simulink model "Model_1_with_driver"  (R2021a)
settings: Solver=VariableStepAuto  StartTime=0.0  StopTime=1561  RelTol=1e-3
model workspace (MATLAB code in the model file):
  | ms = 135;
  | mf = 5;
  | mr = 10;
  | m = ms + (mf + mr);
  | a = 0.7;
  | b = 0.7;
  | Cd = 0.8;
  | Af = 1;
  | h_cg = 0.5;
  | kf = 10000;
  | kr = 15000;
  | cf = 5000;
  | cr = 5000;
  | I = 500;
  | kt = 175000;
  | GR = 6.5;
  | Pmax = 5500;
  | Tmax = 26;
undefined symbols (not defined in the file or in its folder): bev
libraries: fl_lib x9, autolibshared x4, nesl_utility x3
(part 1 of 3)
settings Model: Creator=Barath Krishna S  LastModifiedBy=Ng
settings SolverCC: AlgebraicLoopSolver=TrustRegion
settings DebuggingCC: SFMachineParentedDataDiag=warning

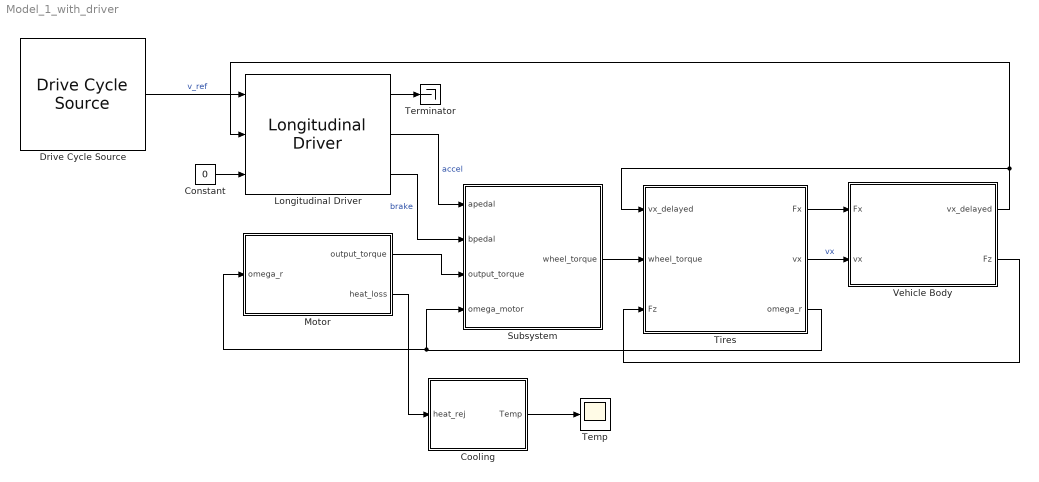
== system Model_1_with_driver ==
  Constant : Constant  Value=0
  Cooling : Subsystem
  Drive Cycle Source : autolibshared/Drive Cycle Source  cycleVar=Workspace variable  wsVar=mycycle  fileVar=cycleFTP75.mat  tfinal="1560.636  seconds"  cycleRepeat=off  outAccPort=off  outGearPort=off  gearList=No gear data  t_wot1=5  xdot_woto=0  xdot_wot1=30  t_wot2=20  xdot_wot2=0  t_wotend=30  srcUnit=m/s  outUnit=m/s  srcAccUnit=m/s/s  outAccUnit=m/s^2  dt=0  aMode=1  faultOption=off  velBnd=2  velBndUnit=mph  inUnit=m/s  timeBnd=1  failOption=off  stopSim=off  maxFaultCnt=10  maxFaultTime=2  maxTotFaultTime=15  traceOption=off  dtTrace=1  traceWindow=10  lastDCname=Custom Data Set  lastOutUnit=mph  lastDT=0  lastTB=1  lastSB=2  forceCalcBound=off
      settings: SourceProductBaseCode=PW,DR,MT,UV,VE
  Longitudinal Driver : autolibshared/Longitudinal Driver  extAccelOvr=off  extDecelOvr=off  extAccelHld=off  extDecelHld=off  extAccelZero=off  extDecelZero=off  cntrlType=PI  shftType=None  velUnits=m/s  gearOut=off  Kp=100  Ki=2.5  Kff=.05  Kg=.01  VehVelVec=[0 100]  KffVec=[.1 .1]  KpVec=[10 10]  KiVec=[5 5]  KgVec=[0 0]  m=1500  Kpt=3000  tau=.1  L=2  aR=200  bR=2.5  cR=.5  g=9.81  vnom=100  Kaw=.1  tauerr=.03  tauPt=2  GearInit=0  tShift=.1  pdlVec=[0.1 0.4 0.5 0.9]  upShftTbl=[-1 12.9375 26.4375 39.9375 51.18749999999999 62.4375 72.84375 83.25;-1 16.3125 29.8125 43.3125 54.5624 65.8125 76.78125 87.75;-1 19.6875 33.1875 46.68749999999999 57.9375 69.1875 80.71875 92.25;-1 33 52.5 77.25 100.5 138.75 161.875 185]  dwnShftTbl=[1 9.5625 23.0625 36.5625 47.8125 59.0625 68.90625 78.75;1 12.9375 26.4375 39.9375 51.18749999999999 62.4375 72.84375 83.25;1 16.3125 29.8125 43.3125 54.562499 65.8125 76.78125 87.75;1 19.6875 33.1875 46.68749999999999 57.9375 69.1875 80.71875 92.25]  tClutch=.5  tRev=.5  tPark=120  aMode=1  UpGearVec="[0  1  2  3  4  5  6  7]"  DownGearVec="[1  2  3  4  5  6  7  8]"
      settings: SourceProductBaseCode=PW,DR,MT,UV,VE
  Motor : Subsystem
  Subsystem : Subsystem
  Temp : Scope
  Terminator : Terminator
  Tires : Subsystem
  Vehicle Body : Subsystem
  wires:
  Tires/2(vx) -> Vehicle Body/2(vx)  "vx"
  Vehicle Body/2(Fz) -> Tires/3(Fz)
  Vehicle Body/1(vx_delayed) -> Longitudinal Driver/2, Tires/1(vx_delayed)
  Tires/1(Fx) -> Vehicle Body/1(Fx)
  Drive Cycle Source/1 -> Longitudinal Driver/1  "v_ref"
  Constant/1 -> Longitudinal Driver/3
  Longitudinal Driver/1 -> Terminator/1
  Longitudinal Driver/2 -> Subsystem/1(apedal)  "accel"
  Longitudinal Driver/3 -> Subsystem/2(bpedal)  "brake"
  Motor/1(output_torque) -> Subsystem/3(output_torque)
  Subsystem/1(wheel_torque) -> Tires/2(wheel_torque)
  Tires/3(omega_r) -> Subsystem/4(omega_motor), Motor/1(omega_r)
  Motor/2(heat_loss) -> Cooling/1(heat_rej)
  Cooling/1(Temp) -> Temp/1

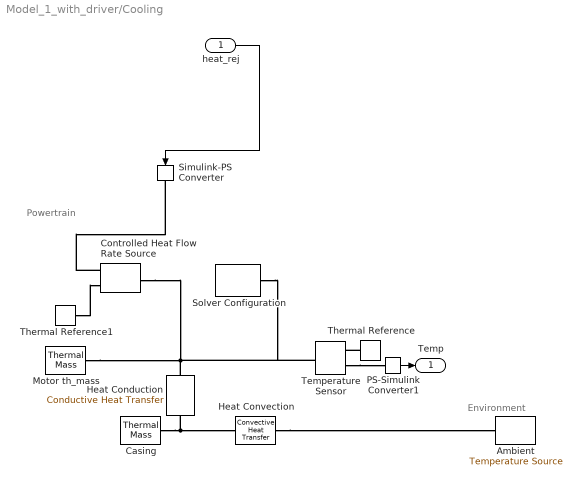
== system Model_1_with_driver/Cooling ==
  note: Powertrain
  note: Environment
  heat_rej : Inport
  Ambient : fl_lib/Thermal/Thermal Sources/Temperature Source  temperature=bev.Tambient degC
  Casing : fl_lib/Thermal/Thermal Elements/Thermal Mass  mass=bev.casing.mass kg  sp_heat=bev.casing.sp_heat J/kg/K  T_specify=on  T_priority=High  T=bev.casing.initT degC  T_nominal_specify=off  T_nominal_unit=K  T_nominal_value=1  Q_specify=off  Q_priority=None  Q=0 W  Q_nominal_specify=off  Q_nominal_unit=W  Q_nominal_value=1
  Controlled Heat Flow Rate Source : fl_lib/Thermal/Thermal Sources/Controlled Heat Flow Rate Source
  Heat Conduction : fl_lib/Thermal/Thermal Elements/Conductive Heat Transfer  area=bev.motor.qcond.area m^2  thickness=bev.motor.qcond.thick m  th_cond=bev.motor.qcond.th_cond W/(m*K)  T_specify=off  T_priority=None  T=0 K  T_nominal_specify=off  T_nominal_unit=K  T_nominal_value=1  Q_specify=off  Q_priority=None  Q=1 W  Q_nominal_specify=off  Q_nominal_unit=W  Q_nominal_value=1
  Heat Convection : fl_lib/Thermal/Thermal Elements/Convective Heat Transfer  area=bev.casing.qconv.area m^2  heat_tr_coeff=bev.casing.qconv.th_conv W/(m^2 * K)  T_specify=off  T_priority=None  T=0 K  T_nominal_specify=off  T_nominal_unit=K  T_nominal_value=1  Q_specify=off  Q_priority=None  Q=0 W  Q_nominal_specify=off  Q_nominal_unit=W  Q_nominal_value=1
  Motor th_mass : fl_lib/Thermal/Thermal Elements/Thermal Mass  mass=bev.motor.thermal_mass kg  sp_heat=1 J/kg/K  T_specify=on  T_priority=High  T=bev.motor.initT degC  T_nominal_specify=off  T_nominal_unit=K  T_nominal_value=1  Q_specify=off  Q_priority=None  Q=0 W  Q_nominal_specify=off  Q_nominal_unit=W  Q_nominal_value=1
  PS-Simulink Converter1 : nesl_utility/PS-Simulink Converter  PhysicalDomain=network_engine_domain  SubClassName=ps_output  LeftPortType=input  RightPortType=output  PseudoPeriodic=off  Frequencies=[]  Unit=degC  AffineConversion=on
      settings: SourceProductBaseCode=PW,SS
  Simulink-PS Converter : nesl_utility/Simulink-PS Converter  PhysicalDomain=network_engine_domain  SubClassName=ps_input  LeftPortType=input  RightPortType=output  PseudoPeriodic=off  Frequencies=[]  NoiseDistribution=none  NoiseParameters=[]  Unit=1  AffineConversion=off  FilteringAndDerivatives=provide  SimscapeFilterOrder=1  InputFilterTimeConstant=0.001  UdotUserProvided=0
      settings: SourceProductBaseCode=PW,SS
  Solver Configuration : nesl_utility/Solver Configuration  PhysicalDomain=network_engine_domain  SubClassName=solver  LeftPortType=input  RightPortType=generic  Tones=[]  Harmonics=[]  SimulateNoise=off  Profile=off  UseLocalSampling=off  EnableSwitchedLinearOptims=on  FrequencyDomain=off  UseCCode=off  RelTol=0.001  AbsTol=1e-06  MinStep=1e-09  ToWorkspace=off  RevertToSquareIcSolve=off  NumHomotopyIterations=100  PhasorMode=off  PhasorModeNumHarmonics=1  DoDC=off  ResidualTolerance=1e-09  UseLocalSolver=off  LocalSolverChoice=NE_BACKWARD_EULER_ADVANCER  LocalSolverSampleTime=0.001  DoFixedCost=off  MaxNonlinIter=3  MaxModeIter=2  ComputeImpulses=off  ImpulseIterations=2  LinearAlgebra=auto  EquationFormulation=NE_TIME_EF  DelaysMemoryBudget=1024  AutomaticFiltering=on  FilteringTimeConstant=0.001  PartitionStorageMethod=AS_NEEDED  PartitionMemoryBudget=1024  PartitionMethod=ROBUST
      settings: SourceProductName=Utilities
  Temperature Sensor : fl_lib/Thermal/Thermal Sensors/Temperature Sensor
  Thermal Reference : fl_lib/Thermal/Thermal Elements/Thermal Reference
  Thermal Reference1 : fl_lib/Thermal/Thermal Elements/Thermal Reference
  Temp : Outport
  wires:
  heat_rej/1 -> Simulink-PS Converter/1
  PS-Simulink Converter1/1 -> Temp/1
  connections:
  Heat Conduction/RConn1 -- Heat Convection/LConn1 -- Casing/LConn1
  Heat Convection/RConn1 -- Ambient/LConn1
  Thermal Reference/LConn1 -- Temperature Sensor/RConn1
  Temperature Sensor/RConn2 -- PS-Simulink Converter1/LConn1
  Heat Conduction/LConn1 -- Controlled Heat Flow Rate Source/LConn1 -- Temperature Sensor/LConn1 -- Solver Configuration/RConn1 -- Motor th_mass/LConn1
  Thermal Reference1/LConn1 -- Controlled Heat Flow Rate Source/RConn2
  Controlled Heat Flow Rate Source/RConn1 -- Simulink-PS Converter/RConn1

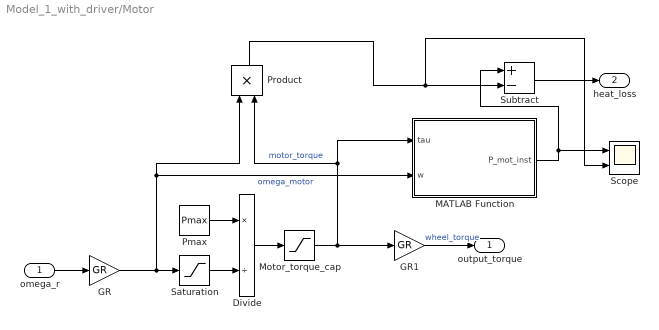
== system Model_1_with_driver/Motor ==
  omega_r : Inport
  Divide : Product  Inputs=*/
  GR : Gain  Gain=GR
  GR1 : Gain  Gain=GR
  MATLAB Function : MATLAB Function  TreatAsAtomicUnit=on
  Motor_torque_cap : Saturate  UpperLimit=Tmax  LowerLimit=0
  Pmax : Constant  Value=Pmax
  Product : Product
  Saturation : Saturate  UpperLimit=inf  LowerLimit=0.001
  Scope : Scope  NumInputPorts=2
  Subtract : Sum  Inputs=+-
  output_torque : Outport
  heat_loss : Outport  Port=2
  wires:
  Pmax/1 -> Divide/1
  Saturation/1 -> Divide/2
  Divide/1 -> Motor_torque_cap/1
  omega_r/1 -> GR/1
  GR1/1 -> output_torque/1  "wheel_torque"
  Subtract/1 -> heat_loss/1
  GR/1 -> Product/1, MATLAB Function/2(w), Saturation/1  "omega_motor"
  Motor_torque_cap/1 -> GR1/1, MATLAB Function/1(tau), Product/2  "motor_torque"
  MATLAB Function/1(P_mot_inst) -> Subtract/1, Scope/1
  Product/1 -> Scope/2, Subtract/2

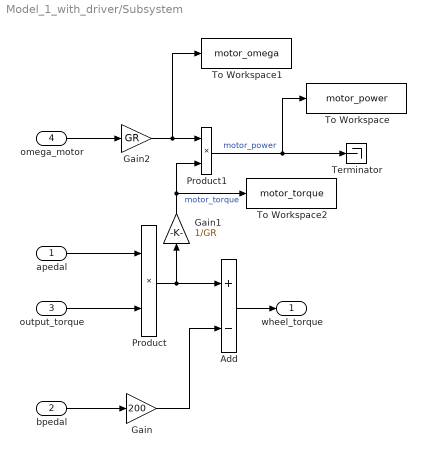
== system Model_1_with_driver/Subsystem ==
  apedal : Inport
  bpedal : Inport  Port=2
  output_torque : Inport  Port=3
  omega_motor : Inport  Port=4
  Add : Sum  Inputs=+-
  Gain : Gain  Gain=200
  Gain1 : Gain  Gain=1/GR
  Gain2 : Gain  Gain=GR
  Product : Product
  Product1 : Product
  Terminator : Terminator
  To Workspace : ToWorkspace  VariableName=motor_power  SampleTime=0.1
  To Workspace1 : ToWorkspace  VariableName=motor_omega  SampleTime=0.1
  To Workspace2 : ToWorkspace  VariableName=motor_torque  SampleTime=0.1
  wheel_torque : Outport
  wires:
  apedal/1 -> Product/1
  output_torque/1 -> Product/2
  bpedal/1 -> Gain/1
  Gain/1 -> Add/2
  Product/1 -> Add/1, Gain1/1
  Add/1 -> wheel_torque/1
  omega_motor/1 -> Gain2/1
  Product1/1 -> Terminator/1, To Workspace/1  "motor_power"
  Gain1/1 -> To Workspace2/1, Product1/2  "motor_torque"
  Gain2/1 -> To Workspace1/1, Product1/1
